simulink model "L0301"  (Simulink 9.1)
settings: Solver=ode45  StartTime=0.0  StopTime=30  MaxStep=0.01  RelTol=1e-3
libraries: simulink x2
settings Model: Creator=Asus  LastModifiedBy=Asus
settings DataIOCC: SaveFormat=Dataset
settings OptimizationCC: LifeSpan=auto
settings DebuggingCC: UnderspecifiedInitializationDetection=Simplified  MergeDetectMultiDrivingBlocksExec=error  SFUnexpectedBacktrackingDiag=error  SFNoUnconditionalDefaultTransitionDiag=error  SFExecutionAtInitializationDiag=warning
settings HardwareCC: ProdBitPerPointer=64  ProdBitPerSizeT=64  ProdBitPerPtrDiffT=64  ProdLargestAtomicFloat=Float  ProdIntDivRoundTo=Zero  ProdEndianess=LittleEndian  ProdWordSize=64  ProdHWDeviceType=Intel->x86-64 (Windows64)
settings ModelReferenceCC: PropagateSignalLabelsOutOfModel=on
settings CodeAppCC: StateflowObjectComments=off
settings GRTTargetCC: TargetLangStandard=C99 (ISO)  CombineOutputUpdateFcns=on  GRTInterface=off
settings ConfigComp: CovMetricSettings=dwe  CovHtmlReporting=off  CovSaveCumulativeToWorkspaceVar=off  CovSaveSingleToWorkspaceVar=off  CovExternalEMLEnable=on

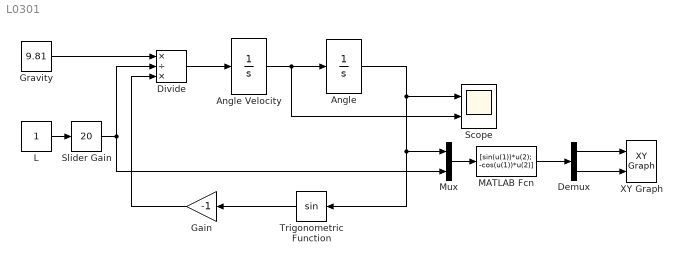
== system L0301 ==
  Angle : Integrator
  Angle Velocity : Integrator  InitialCondition=2
  Demux : Demux  Outputs=2
  Divide : Product  Inputs=*/*
  Gain : Gain  Gain=-1
  Gravity : Constant  Value=9.81
  L : Constant
  MATLAB Fcn : MATLABFcn  MATLABFcn=[sin(u(1))*u(2); -cos(u(1))*u(2)]
  Mux : Mux  Inputs=2
  Scope : Scope  NumInputPorts=2
  Slider Gain : simulink/Math Operations/Slider Gain  gain=20  low=0  high=50
  Trigonometric Function : Trigonometry
  XY Graph : simulink/Sinks/XY Graph  xmin=-35  xmax=35  ymin=-35  ymax=35  st=-1
  wires:
  MATLAB Fcn/1 -> Demux/1
  Angle/1 -> Trigonometric Function/1, Mux/1, Scope/1
  Angle Velocity/1 -> Angle/1, Scope/2
  Demux/2 -> XY Graph/2
  Demux/1 -> XY Graph/1
  Mux/1 -> MATLAB Fcn/1
  Gravity/1 -> Divide/1
  Slider Gain/1 -> Divide/2, Mux/2
  Trigonometric Function/1 -> Gain/1
  Gain/1 -> Divide/3
  Divide/1 -> Angle Velocity/1
  L/1 -> Slider Gain/1
